simulink model "pendulo_nao_linear"  (R2020b)
settings: Solver=FixedStepAuto  StartTime=0.0  StopTime=10  FixedStep=1e-3  RelTol=1e-3
values from neighbouring files (symbols this model uses):
  controlador = projetarControlador(requisitos, planta)    [executarTudo.m]    (also in runAll.m)
  model = obterParametros(planta, varianciaComando, varianciaMedida)    [executarTudo.m]    (also in runAll.m = getParameters(planta, varCom, varMed))
  planta = obterPlanta()    [codetest.m]    (also in executarTudo.m; nextState.m; runAll.m)
  thetar = 0    [executarTudo.m]    (also in runAll.m = 0.1)
  varCom = 0.001    [runAll.m]
  varMed = 0.001    [runAll.m]
libraries: pid_lib x1
settings Model: Creator=davi  LastModifiedBy=alexandremaranhao

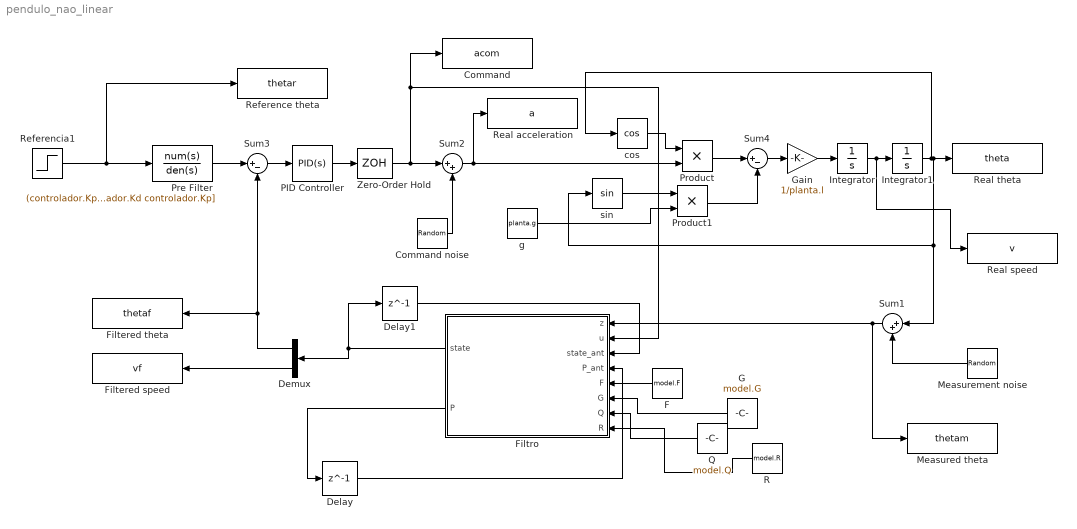
== system pendulo_nao_linear ==
  Command : ToWorkspace  VariableName=acom  SaveFormat=Structure With Time  SampleTime=-1
  Command noise : RandomNumber  Variance=varCom  SampleTime=1e-2
  Delay : Delay  DelayLength=1  InitialCondition=eye(2)  SampleTime=1e-2
  Delay1 : Delay  DelayLength=1  InitialCondition=[0;0]  SampleTime=1e-2
  Demux : Demux  Outputs=2
  F : Constant  Value=model.F
  Filtered speed : ToWorkspace  VariableName=vf  SaveFormat=Structure With Time  SampleTime=-1
  Filtered theta : ToWorkspace  VariableName=thetaf  SaveFormat=Structure With Time  SampleTime=-1
  Filtro : MATLAB Function  TreatAsAtomicUnit=on  SystemSampleTime=1e-2
  G : Constant  Value=model.G
  Gain : Gain  Gain=1/planta.l
  Integrator : Integrator
  Integrator1 : Integrator
  Measured theta : ToWorkspace  VariableName=thetam  SaveFormat=Structure With Time  SampleTime=-1
  Measurement noise : RandomNumber  Variance=varMed  SampleTime=1e-2
  PID Controller : pid_lib/PID Controller  Controller=PID  Form=Parallel  TimeDomain=Continuous-time  UseExternalTs=off  SampleTime=1e-2  IntegratorMethod=Forward Euler  FilterMethod=Forward Euler  ControllerParametersSource=internal  P=controlador.Kp  I=0  D=controlador.Kd  UseFilter=on  N=100  TunerSelectOption=Transfer Function Based (PID Tuner App)  InitialConditionSource=internal  InitialConditionForIntegrator=0  InitialConditionForFilter=0  DifferentiatorICPrevScaledInput=0  ExternalReset=none  TrackingMode=off  Kt=1  LimitOutput=off  SatLimitsSource=internal  UpperSaturationLimit=inf  LowerSaturationLimit=-inf  LinearizeAsGain=on  AntiWindupMode=none  Kb=1  POutMin=[]  POutMax=[]  IOutMin=[]  IOutMax=[]  DOutMin=[]  DOutMax=[]  NOutMin=[]  NOutMax=[]  SumOutMin=[]  SumOutMax=[]  SaturationOutMin=[]  SaturationOutMax=[]  PParamMin=[]  PParamMax=[]  IParamMin=[]  IParamMax=[]  DParamMin=[]  DParamMax=[]  NParamMin=[]  NParamMax=[]  KbParamMin=[]  KbParamMax=[]  KtParamMin=[]  KtParamMax=[]  KbOutMin=[]  KbOutMax=[]  KtOutMin=[]  KtOutMax=[]  IntegratorOutMin=[]  IntegratorOutMax=[]  FilterOutMin=[]  FilterOutMax=[]  SumI1OutMin=[]  SumI1OutMax=[]  SumI2OutMin=[]  SumI2OutMax=[]  SumI3OutMin=[]  SumI3OutMax=[]  SumI4OutMin=[]  SumI4OutMax=[]  SumDOutMin=[]  SumDOutMax=[]  DifferentiatorOutMin=[]  DifferentiatorOutMax=[]  FilterDiffOutCoefMin=[]  FilterDiffOutCoefMax=[]  ReciprocalOutMin=[]  ReciprocalOutMax=[]  SumDenOutMin=[]  SumDenOutMax=[]  SumNumOutMin=[]  SumNumOutMax=[]  DivideOutMin=[]  DivideOutMax=[]  UdiffTsProdOutMin=[]  UdiffTsProdOutMax=[]  NTsProdOutMin=[]  NTsProdOutMax=[]  UintegralTsProdOutMin=[]  UintegralTsProdOutMax=[]  UngainTsProdOutMin=[]  UngainTsProdOutMax=[]  IntegratorContinuousStateAttributes=''  IntegratorStateMustResolveToSignalObject=off  IntegratorRTWStateStorageClass=Auto  FilterContinuousStateAttributes=''  FilterStateMustResolveToSignalObject=off  FilterRTWStateStorageClass=Auto  ParallelPVariant=InternalParameters  IdealPVariant=Disabled  IVariant=InternalParameters  DVariant=InternalParameters  IntegratorVariant=Continuous  SatVariant=Disabled  AWVariant=Passthrough  PCopyVariant=Disabled  TRVariant=Disabled  FdbkBlocksVariant=Forward  IdealPFdbkVariant=Disabled  SatFdbkVariant=Disabled  DerivativeFilterVariant=ContFilter  NVariant=InternalParameters  NCopyVariant=Disabled  FilterICVariant=InternalICsFilter  IntegratorICVariant=InternalICs  ExternalResetVariant=Disabled  TRSumVariant=Passthrough  SumFdbkVariant=Disabled  SumVariant=Sum_PID  TsampFilterVariant=InternalTs  TsampNgainVariant=Passthrough  TsampIntegralVariant=Passthrough  ExternalSaturationOutDataTypeStr=Inherit: Same as second input
  Pre Filter : TransferFcn  Numerator=(controlador.Kp+planta.g)  Denominator=[controlador.Kd controlador.Kp]
  Product : Product
  Product1 : Product
  Q : Constant  Value=model.Q
  R : Constant  Value=model.R
  Real acceleration : ToWorkspace  VariableName=a  SaveFormat=Structure With Time  SampleTime=-1
  Real speed : ToWorkspace  VariableName=v  SaveFormat=Structure With Time  SampleTime=-1
  Real theta : ToWorkspace  VariableName=theta  SaveFormat=Structure With Time  SampleTime=-1
  Reference theta : ToWorkspace  VariableName=thetar  SaveFormat=Structure With Time  SampleTime=-1
  Referencia1 : Step  Time=0  After=thetar  SampleTime=0
  Sum1 : Sum  Inputs=|++
  Sum2 : Sum  Inputs=|++
  Sum3 : Sum  Inputs=|+-
  Sum4 : Sum  Inputs=|+-
  Zero-Order Hold : ZeroOrderHold  SampleTime=1e-2
  cos : Trigonometry  Operator=cos
  g : Constant  Value=planta.g
  sin : Trigonometry
  wires:
  Product/1 -> Sum4/1
  Measurement noise/1 -> Sum1/2
  Sum2/1 -> Product/2, Real acceleration/1
  Command noise/1 -> Sum2/2
  Referencia1/1 -> Pre Filter/1, Reference theta/1
  Pre Filter/1 -> Sum3/1
  cos/1 -> Product/1
  sin/1 -> Product1/1
  g/1 -> Product1/2
  Product1/1 -> Sum4/2
  Sum4/1 -> Gain/1
  Gain/1 -> Integrator/1
  Integrator/1 -> Real speed/1, Integrator1/1
  Integrator1/1 -> sin/1, Sum1/1, Real theta/1, cos/1
  Sum3/1 -> PID Controller/1
  Sum1/1 -> Measured theta/1, Filtro/1(z)
  Filtro/1(state) -> Delay1/1, Demux/1
  Filtro/2(P) -> Delay/1
  Delay1/1 -> Filtro/3(state_ant)
  Delay/1 -> Filtro/4(P_ant)
  Demux/2 -> Filtered speed/1
  Demux/1 -> Sum3/2, Filtered theta/1
  PID Controller/1 -> Zero-Order Hold/1
  Zero-Order Hold/1 -> Filtro/2(u), Command/1, Sum2/1
  F/1 -> Filtro/5(F)
  G/1 -> Filtro/6(G)
  Q/1 -> Filtro/7(Q)
  R/1 -> Filtro/8(R)

== matlab function pendulo_nao_linear/Filtro ==
  settings: updateMethod=DISCRETE
  data: state output; z input; u input; state_ant input; P_ant input; P output; F input; G input; Q input; R input
function [state, P] = fcn(z, u, state_ant, P_ant, F, G, Q, R)

x_pred = F*state_ant + G*u;
P_pred = F*P_ant*F' + Q;

C = [1 0];
Kt = P_pred * C' * pinv(R + C*P_pred*C');
state = x_pred + Kt*(z-C*state_ant);
P = P_pred - Kt*C*P_pred;

end
